simulink model "AOO_Draft"  (R2022b)
settings: Solver=FixedStepAuto  StartTime=0.0  StopTime=10.0  FixedStep=1e-3  RelTol=1e-3  EnableMultiTasking=on
undefined symbols (not defined in the file): D10, D11, D12, D2, D4, D5, D7, D8, D9, PTA0, PTA2, PTB23, PTB9, PTC3, PTC4, PTD0, PTD2, PTD3
libraries: frdmk64flib x9
settings Model: ExtModeTrigDuration=5  Creator=Mehak  LastModifiedBy=Mehak
settings OptimizationCC: EnhancedBackFolding=on  PassReuseOutputArgsAs=Individual arguments  ZeroExternalMemoryAtStartup=off  ZeroInternalMemoryAtStartup=off  MaxStackSize=64  OptimizeBlockOrder=speed  DifferentSizesBufferReuse=on  OptimizationCustomize=off  EfficientTunableParamExpr=on
settings DebuggingCC: ParameterTunabilityLossMsg=error
settings HardwareCC: ProdBitPerPointer=32  ProdBitPerSizeT=32  ProdBitPerPtrDiffT=32  ProdLargestAtomicInteger=Long  ProdLargestAtomicFloat=Double  ProdWordSize=32  ProdHWDeviceType=ARM Compatible->ARM Cortex
settings SFSimCC: MATLABDynamicMemAlloc=off
settings RTWCC: Description=Embedded Coder  SystemTargetFile=ert.tlc  HardwareBoard=NXP FRDM-K64F  TLCOptions="-aInlineSetEventsForThisBaseRateFcn=TLC_FALSE -aSuppressMultiTaskScheduler=TLC_FALSE  -aRateBasedStepFcn=0"  TemplateMakefile=ert_default_tmf  Toolchain=GNU Tools for ARM Embedded Processors
settings CodeAppCC: ForceParamTrailComments=on  IgnoreCustomStorageClasses=off  OperatorAnnotations=on  SimulinkDataObjDesc=on  SFDataObjDesc=on  InsertBlockDesc=on
settings ERTTargetCC: ExtModeTransport=4  ExtModeMexFile=sendToCommService

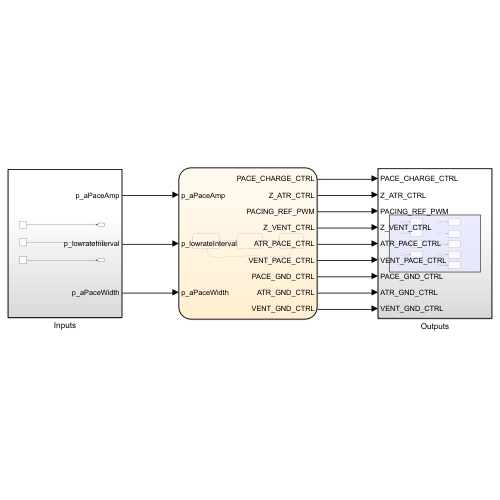
[thumbnail: Simulink's stored preview of the top-level diagram]
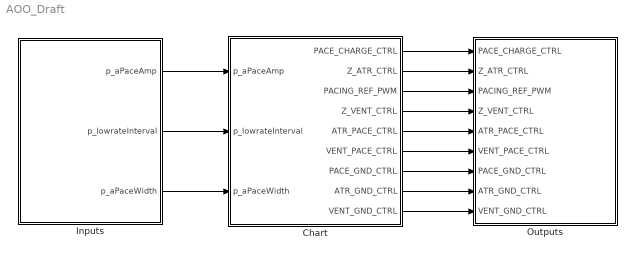
== system AOO_Draft ==
  Chart : Stateflow chart  TreatAsAtomicUnit=on
      settings: PortSchema="{\"entries\":[{\"content\":{\"sides\":[{\"content\":{\"connectorIds\":[\"In2\",\"In1\",\"In3\"]},\"type\":\"ConnectorPlacement.EquallySpacedRectSide\",\"uuid\":\"98db9cea-c46a-4cd8-8963-54ca314d30e1\"},{\"content\":{\"connectorIds\":[\"Out1\",\"Out2\",\"Out3\",\"Out4\",\"Out5\",\"Out6\",\"Out7\",\"Out8\",\"Out9\"],\"side\":\"RIGHT\"},\"type\":\"ConnectorPlacement.EquallySpacedRectSide\",\"uuid\":\"53c86289-975b-4bf4-bda6-3305a5df9915\"},{\"content\":{\"connectorIds\":[],\"side\":\"TOP\"},\"type\":\"ConnectorPlacement.EquallySpacedRectSide\",\"uuid\":\"435718e2-c076-4bdf-bdcc-26eba696f870\"}]},\"type\":\"ConnectorPlacement.EquallySpacedConnector\",\"uuid\":\"74f4dc21-b756-4a46-a28e-6c66b22264cf\"}],\"packageUris\":[\"http://schema.mathworks.com/mf0/Connector/R2020b\"],\"version\":\"1.0\"}"
  Inputs : Subsystem
  Outputs : Subsystem
  wires:
  Chart/1(PACE_CHARGE_CTRL) -> Outputs/1(PACE_CHARGE_CTRL)
  Chart/2(Z_ATR_CTRL) -> Outputs/2(Z_ATR_CTRL)
  Chart/3(PACING_REF_PWM) -> Outputs/3(PACING_REF_PWM)
  Chart/4(Z_VENT_CTRL) -> Outputs/4(Z_VENT_CTRL)
  Chart/5(ATR_PACE_CTRL) -> Outputs/5(ATR_PACE_CTRL)
  Chart/7(PACE_GND_CTRL) -> Outputs/7(PACE_GND_CTRL)
  Chart/6(VENT_PACE_CTRL) -> Outputs/6(VENT_PACE_CTRL)
  Chart/9(VENT_GND_CTRL) -> Outputs/9(VENT_GND_CTRL)
  Chart/8(ATR_GND_CTRL) -> Outputs/8(ATR_GND_CTRL)
  Inputs/1(p_aPaceAmp) -> Chart/2(p_aPaceAmp)
  Inputs/2(p_lowrateInterval) -> Chart/1(p_lowrateInterval)
  Inputs/3(p_aPaceWidth) -> Chart/3(p_aPaceWidth)

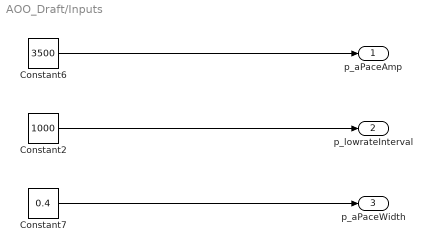
== system AOO_Draft/Inputs ==
  Constant2 : Constant  Value=1000
  Constant6 : Constant  Value=3500
  Constant7 : Constant  Value=0.4
  p_aPaceAmp : Outport
  p_lowrateInterval : Outport  Port=2
  p_aPaceWidth : Outport  Port=3
  wires:
  Constant6/1 -> p_aPaceAmp/1
  Constant2/1 -> p_lowrateInterval/1
  Constant7/1 -> p_aPaceWidth/1

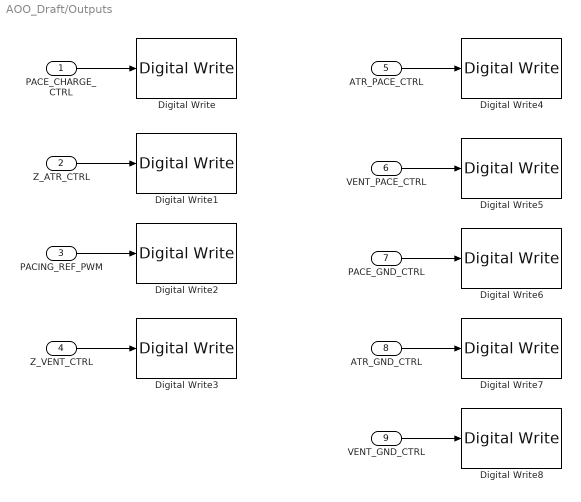
== system AOO_Draft/Outputs ==
  PACE_CHARGE_CTRL : Inport
  Z_ATR_CTRL : Inport  Port=2
  PACING_REF_PWM : Inport  Port=3
  Z_VENT_CTRL : Inport  Port=4
  ATR_PACE_CTRL : Inport  Port=5
  VENT_PACE_CTRL : Inport  Port=6
  PACE_GND_CTRL : Inport  Port=7
  ATR_GND_CTRL : Inport  Port=8
  VENT_GND_CTRL : Inport  Port=9
  Digital Write : frdmk64flib/Digital Write  Whichpin=PTB9 (D2)
  Digital Write1 : frdmk64flib/Digital Write  Whichpin=PTB23 (D4)
  Digital Write2 : frdmk64flib/Digital Write  Whichpin=PTA2 (D5)
  Digital Write3 : frdmk64flib/Digital Write  Whichpin=PTC3 (D7)
  Digital Write4 : frdmk64flib/Digital Write  Whichpin=PTA0 (D8)
  Digital Write5 : frdmk64flib/Digital Write  Whichpin=PTC4 (D9)
  Digital Write6 : frdmk64flib/Digital Write  Whichpin=PTD0 (D10)
  Digital Write7 : frdmk64flib/Digital Write  Whichpin=PTD2 (D11)
  Digital Write8 : frdmk64flib/Digital Write  Whichpin=PTD3 (D12)
  wires:
  PACE_CHARGE_CTRL/1 -> Digital Write/1
  Z_ATR_CTRL/1 -> Digital Write1/1
  PACING_REF_PWM/1 -> Digital Write2/1
  Z_VENT_CTRL/1 -> Digital Write3/1
  ATR_PACE_CTRL/1 -> Digital Write4/1
  PACE_GND_CTRL/1 -> Digital Write6/1
  VENT_PACE_CTRL/1 -> Digital Write5/1
  VENT_GND_CTRL/1 -> Digital Write8/1
  ATR_GND_CTRL/1 -> Digital Write7/1

== stateflow chart AOO_Draft/Chart ==
  state Charging
    entry:
    ATR_PACE_CTRL = 0;
    VENT_PACE_CTRL = 0;
    PACING_REF_PWM = ((p_aPaceAmp)/10)/5;
    PACE_CHARGE_CTRL = 1;
  state Pacing
    entry:
    PACE_CHARGE_CTRL = 0;
    PACE_GND_CTRL = 1;
    ATR_PACE_CTRL = 1;
    ATR_GND_CTRL = 0;
    Z_ATR_CTRL = 0;
    Z_VENT_CTRL = 0;
    VENT_GND_CTRL = 0;
    VENT_PACE_CTRL = 0;
  state Discharging
    entry:
    PACE_GND_CTRL = 1;
    VENT_PACE_CTRL = 0;
    Z_ATR_CTRL = 0;
    Z_VENT_CTRL = 0;
    ATR_PACE_CTRL = 0;
    ATR_GND_CTRL = 1;
    VENT_GND_CTRL = 0;
  (default) -> Charging
  Pacing -> Discharging : after(p_aPaceWidth, msec)
  Charging -> Pacing : after(p_lowrateInterval, msec)
  Discharging -> Charging
  data: PACE_CHARGE_CTRL output int16; Z_ATR_CTRL output int16; PACING_REF_PWM output double; Z_VENT_CTRL output int16; ATR_PACE_CTRL output int16; VENT_PACE_CTRL output int16; PACE_GND_CTRL output int16; ATR_GND_CTRL output int16; VENT_GND_CTRL output int16; p_lowrateInterval input double; p_aPaceAmp input double; p_aPaceWidth input
